simulink library "SUB_ECU_L4_MABX_HW_Interface"  (R2018a)
settings: Solver=VariableStepAuto  StartTime=0.0  StopTime=10.0  RelTol=1e-3
PostLoadFcn:
  | , if any(exist('dsrtsu_mdlpostloadfcn', 'file') == [2, 3, 6]), try dsrtsu_mdlpostloadfcn('Execute', bdroot); catch fprintf('Error in PostLoadFcn (dsrtsu_mdlpostloadfcn) for model "%s":\n %s\n', bdroot, lasterr); end, end,
undefined symbols (not defined in the file or in its folder): CANR_PROPB_REAX_3_13_CHANNEL_APV, CANR_PROPB_REAX_4_13_CHANNEL_APV, CANR_PROPB_XPR_1_50_CHANNEL_APV, ENUM_CAN_RX_T, ENUM_CAN_TX_T, ENUM_REAX_OPERATION_MODE_T, ENUM_SIGNAL_HEALTH_T, ENUM_XBR_CONTROL_MODE_T, ENUM_XBR_EBI_MODE_T, ENUM_XBR_PASS_THROUGH_ACTIVE_T, ENUM_XBR_PRIORITY_T, ENUM_XPR_INHIBIT_PARK_MANUAL_T, ENUM_XPR_INHIBIT_UNPARK_MANUAL_T, ENUM_XPR_PARK_MANUAL_T, ENUM_XPR_UNPARK_MANUAL_T, PROPB_REAX_1_E4_DES_POS_SIG_SRC_APV, PROPB_REAX_1_E4_DESIRED_OPMODE_APV, PROPB_REAX_1_E4_DESIRED_POSITION_APV, ptc_matlab_lib
libraries: PTC_MBDS_LIB x264, rtican x172, EmE_MBD_Blockset x39, simulink x34, $bdroot x16, rti1401lib_dio_type4 x8, simulink_need_slupdate x7, dsa_tcpip_lib x4, rti1401lib_adc_type4 x3, rtmapslib x3, rtitasklib x3
(part 51 of 51)

== system SUB_ECU_L4_MABX_HW_Interface/DIGITAL/PWM pedal input management/Diagnose pedal input signals/Leaky_bucket1 ==
  Signal_valid_range_max : Inport
  Signal_valid_range_min : Inport  Port=2
  Count_Max : Inport  Port=3
  Count_Min : Inport  Port=4
  Input_signal : Inport  Port=5
  Check Dynamic Range1 : simulink/Model Verification/Check  Dynamic Range  Description=min < u < max  enabled=on  stopWhenAssertionFail=off  export=on  icon=graphic
      settings: SourceProductName=Simulink  SourceProductBaseCode=SL
  Decrement Real World3 : simulink/Additional Math & Discrete/Additional Math: Increment - Decrement/Decrement Real World
      settings: SourceProductName=Simulink  SourceProductBaseCode=SL
  Dynamic_saturation3 : EmE_MBD_Blockset/Discontinuities/Dynamic_saturation
      settings: SourceProductName=PACCAR EmE MBD Blockset
  If_Then_Else3 : EmE_MBD_Blockset/Signal Routing/If_Then_Else
      settings: SourceProductName=PACCAR EmE MBD Blockset
  Increment Real World3 : simulink/Additional Math & Discrete/Additional Math: Increment - Decrement/Increment Real World
      settings: SourceProductName=Simulink  SourceProductBaseCode=SL
  Relational Operator8 : RelationalOperator  Operator=<=  OutDataTypeStr=boolean  RndMeth=Nearest
  Relational Operator9 : RelationalOperator  Operator=~=  OutDataTypeStr=boolean  RndMeth=Nearest
  Unit Delay External IC3 : simulink_need_slupdate/Unit Delay External IC  tsamp=-1
      settings: SourceProductName=Simulink  SourceProductBaseCode=SL
  Fault_Count : Outport
  F_Fault_Soft : Outport  Port=2
  F_Fault_Hard : Outport  Port=3
  wires:
  Count_Min/1 -> Unit Delay External IC3/2, Relational Operator9/2, Dynamic_saturation3/3
  Dynamic_saturation3/1 -> Relational Operator9/1, Unit Delay External IC3/1, Fault_Count/1, Relational Operator8/2  "Fault_Count"
  Decrement Real World3/1 -> If_Then_Else3/2
  Increment Real World3/1 -> If_Then_Else3/3
  Relational Operator9/1 -> F_Fault_Soft/1  "F_Fault_Soft"
  Input_signal/1 -> Check Dynamic Range1/3
  Unit Delay External IC3/1 -> Increment Real World3/1, Decrement Real World3/1
  Count_Max/1 -> Relational Operator8/1, Dynamic_saturation3/1
  Relational Operator8/1 -> F_Fault_Hard/1  "F_Fault_Hard"
  Signal_valid_range_max/1 -> Check Dynamic Range1/1
  Check Dynamic Range1/1 -> If_Then_Else3/1  "f_signal_valid"
  Signal_valid_range_min/1 -> Check Dynamic Range1/2
  If_Then_Else3/1 -> Dynamic_saturation3/2

== system SUB_ECU_L4_MABX_HW_Interface/DIGITAL/PWM pedal input management/Diagnose pedal input signals/Leaky_bucket2 ==
  Signal_valid_range_max : Inport
  Signal_valid_range_min : Inport  Port=2
  Count_Max : Inport  Port=3
  Count_Min : Inport  Port=4
  Input_signal : Inport  Port=5
  Check Dynamic Range1 : simulink/Model Verification/Check  Dynamic Range  Description=min < u < max  enabled=on  stopWhenAssertionFail=off  export=on  icon=graphic
      settings: SourceProductName=Simulink  SourceProductBaseCode=SL
  Decrement Real World3 : simulink/Additional Math & Discrete/Additional Math: Increment - Decrement/Decrement Real World
      settings: SourceProductName=Simulink  SourceProductBaseCode=SL
  Dynamic_saturation3 : EmE_MBD_Blockset/Discontinuities/Dynamic_saturation
      settings: SourceProductName=PACCAR EmE MBD Blockset
  If_Then_Else3 : EmE_MBD_Blockset/Signal Routing/If_Then_Else
      settings: SourceProductName=PACCAR EmE MBD Blockset
  Increment Real World3 : simulink/Additional Math & Discrete/Additional Math: Increment - Decrement/Increment Real World
      settings: SourceProductName=Simulink  SourceProductBaseCode=SL
  Relational Operator8 : RelationalOperator  Operator=<=  OutDataTypeStr=boolean  RndMeth=Nearest
  Relational Operator9 : RelationalOperator  Operator=~=  OutDataTypeStr=boolean  RndMeth=Nearest
  Unit Delay External IC3 : simulink_need_slupdate/Unit Delay External IC  tsamp=-1
      settings: SourceProductName=Simulink  SourceProductBaseCode=SL
  Fault_Count : Outport
  F_Fault_Soft : Outport  Port=2
  F_Fault_Hard : Outport  Port=3
  wires:
  Count_Min/1 -> Unit Delay External IC3/2, Relational Operator9/2, Dynamic_saturation3/3
  Dynamic_saturation3/1 -> Relational Operator9/1, Unit Delay External IC3/1, Fault_Count/1, Relational Operator8/2  "Fault_Count"
  Decrement Real World3/1 -> If_Then_Else3/2
  Increment Real World3/1 -> If_Then_Else3/3
  Relational Operator9/1 -> F_Fault_Soft/1  "F_Fault_Soft"
  Input_signal/1 -> Check Dynamic Range1/3
  Unit Delay External IC3/1 -> Increment Real World3/1, Decrement Real World3/1
  Count_Max/1 -> Relational Operator8/1, Dynamic_saturation3/1
  Relational Operator8/1 -> F_Fault_Hard/1  "F_Fault_Hard"
  Signal_valid_range_max/1 -> Check Dynamic Range1/1
  Check Dynamic Range1/1 -> If_Then_Else3/1  "f_signal_valid"
  Signal_valid_range_min/1 -> Check Dynamic Range1/2
  If_Then_Else3/1 -> Dynamic_saturation3/2

== system SUB_ECU_L4_MABX_HW_Interface/DIGITAL/PWM pedal input management/Diagnose pedal input signals/Leaky_bucket3 ==
  Signal_valid_range_max : Inport
  Signal_valid_range_min : Inport  Port=2
  Count_Max : Inport  Port=3
  Count_Min : Inport  Port=4
  Input_signal : Inport  Port=5
  Check Dynamic Range1 : simulink/Model Verification/Check  Dynamic Range  Description=min < u < max  enabled=on  stopWhenAssertionFail=off  export=on  icon=graphic
      settings: SourceProductName=Simulink  SourceProductBaseCode=SL
  Decrement Real World3 : simulink/Additional Math & Discrete/Additional Math: Increment - Decrement/Decrement Real World
      settings: SourceProductName=Simulink  SourceProductBaseCode=SL
  Dynamic_saturation3 : EmE_MBD_Blockset/Discontinuities/Dynamic_saturation
      settings: SourceProductName=PACCAR EmE MBD Blockset
  If_Then_Else3 : EmE_MBD_Blockset/Signal Routing/If_Then_Else
      settings: SourceProductName=PACCAR EmE MBD Blockset
  Increment Real World3 : simulink/Additional Math & Discrete/Additional Math: Increment - Decrement/Increment Real World
      settings: SourceProductName=Simulink  SourceProductBaseCode=SL
  Relational Operator8 : RelationalOperator  Operator=<=  OutDataTypeStr=boolean  RndMeth=Nearest
  Relational Operator9 : RelationalOperator  Operator=~=  OutDataTypeStr=boolean  RndMeth=Nearest
  Unit Delay External IC3 : simulink_need_slupdate/Unit Delay External IC  tsamp=-1
      settings: SourceProductName=Simulink  SourceProductBaseCode=SL
  Fault_Count : Outport
  F_Fault_Soft : Outport  Port=2
  F_Fault_Hard : Outport  Port=3
  wires:
  If_Then_Else3/1 -> Dynamic_saturation3/2
  Signal_valid_range_min/1 -> Check Dynamic Range1/2
  Check Dynamic Range1/1 -> If_Then_Else3/1  "f_signal_valid"
  Signal_valid_range_max/1 -> Check Dynamic Range1/1
  Relational Operator8/1 -> F_Fault_Hard/1  "F_Fault_Hard"
  Count_Max/1 -> Dynamic_saturation3/1, Relational Operator8/1
  Unit Delay External IC3/1 -> Decrement Real World3/1, Increment Real World3/1
  Input_signal/1 -> Check Dynamic Range1/3
  Relational Operator9/1 -> F_Fault_Soft/1  "F_Fault_Soft"
  Increment Real World3/1 -> If_Then_Else3/3
  Decrement Real World3/1 -> If_Then_Else3/2
  Dynamic_saturation3/1 -> Relational Operator8/2, Fault_Count/1, Unit Delay External IC3/1, Relational Operator9/1  "Fault_Count"
  Count_Min/1 -> Dynamic_saturation3/3, Relational Operator9/2, Unit Delay External IC3/2

== system SUB_ECU_L4_MABX_HW_Interface/DIGITAL/PWM pedal input management/Diagnose pedal input signals/Leaky_bucket4 ==
  Signal_valid_range_max : Inport
  Signal_valid_range_min : Inport  Port=2
  Count_Max : Inport  Port=3
  Count_Min : Inport  Port=4
  Input_signal : Inport  Port=5
  Check Dynamic Range1 : simulink/Model Verification/Check  Dynamic Range  Description=min < u < max  enabled=on  stopWhenAssertionFail=off  export=on  icon=graphic
      settings: SourceProductName=Simulink  SourceProductBaseCode=SL
  Decrement Real World3 : simulink/Additional Math & Discrete/Additional Math: Increment - Decrement/Decrement Real World
      settings: SourceProductName=Simulink  SourceProductBaseCode=SL
  Dynamic_saturation3 : EmE_MBD_Blockset/Discontinuities/Dynamic_saturation
      settings: SourceProductName=PACCAR EmE MBD Blockset
  If_Then_Else3 : EmE_MBD_Blockset/Signal Routing/If_Then_Else
      settings: SourceProductName=PACCAR EmE MBD Blockset
  Increment Real World3 : simulink/Additional Math & Discrete/Additional Math: Increment - Decrement/Increment Real World
      settings: SourceProductName=Simulink  SourceProductBaseCode=SL
  Relational Operator8 : RelationalOperator  Operator=<=  OutDataTypeStr=boolean  RndMeth=Nearest
  Relational Operator9 : RelationalOperator  Operator=~=  OutDataTypeStr=boolean  RndMeth=Nearest
  Unit Delay External IC3 : simulink_need_slupdate/Unit Delay External IC  tsamp=-1
      settings: SourceProductName=Simulink  SourceProductBaseCode=SL
  Fault_Count : Outport
  F_Fault_Soft : Outport  Port=2
  F_Fault_Hard : Outport  Port=3
  wires:
  If_Then_Else3/1 -> Dynamic_saturation3/2
  Signal_valid_range_min/1 -> Check Dynamic Range1/2
  Check Dynamic Range1/1 -> If_Then_Else3/1  "f_signal_valid"
  Signal_valid_range_max/1 -> Check Dynamic Range1/1
  Relational Operator8/1 -> F_Fault_Hard/1  "F_Fault_Hard"
  Count_Max/1 -> Dynamic_saturation3/1, Relational Operator8/1
  Unit Delay External IC3/1 -> Decrement Real World3/1, Increment Real World3/1
  Input_signal/1 -> Check Dynamic Range1/3
  Relational Operator9/1 -> F_Fault_Soft/1  "F_Fault_Soft"
  Increment Real World3/1 -> If_Then_Else3/3
  Decrement Real World3/1 -> If_Then_Else3/2
  Dynamic_saturation3/1 -> Relational Operator8/2, Fault_Count/1, Unit Delay External IC3/1, Relational Operator9/1  "Fault_Count"
  Count_Min/1 -> Dynamic_saturation3/3, Relational Operator9/2, Unit Delay External IC3/2

== system SUB_ECU_L4_MABX_HW_Interface/CAN_Out_PTC_1571/CAN_TX_10ms/Encode_PROPB_REAX_1/PropB_REAX_1_E4_CommandFromExternalController/ALL_CTRL_DISABLED ==
  Enable : EnablePort
      settings: AttributesFormatString=States when enabling: %<StatesWhenEnabling>
  Constant : Constant  Value=typecast(uint32(hex2dec('FFFFFFFF')), 'int32')
  Out1 : Outport  InitialOutput=0
      settings: AttributesFormatString=Output when disabled: %<OutputWhenDisabled>
  wires:
  Constant/1 -> Out1/1

== system SUB_ECU_L4_MABX_HW_Interface/CAN_Out_PTC_1571/CAN_TX_10ms/Encode_PROPB_REAX_1/PropB_REAX_1_E4_CommandFromExternalController/DEFAULT_TRQ_CTRL_MODE ==
  Enable : EnablePort
      settings: AttributesFormatString=States when enabling: %<StatesWhenEnabling>
  Constant : Constant  Value=typecast(uint32(hex2dec('FFFFFFFF')), 'int32')
  Out1 : Outport  InitialOutput=0
      settings: AttributesFormatString=Output when disabled: %<OutputWhenDisabled>
  wires:
  Constant/1 -> Out1/1

== system SUB_ECU_L4_MABX_HW_Interface/CAN_Out_PTC_1571/CAN_TX_10ms/Encode_PROPB_REAX_1/PropB_REAX_1_E4_CommandFromExternalController/Desired_Steering_Angle ==
  DesiredSteeringAngle : Inport
  OperatorEnable : Inport  Port=2
  Constant1 : Constant  Value=PROPB_REAX_1_E4_DES_POS_SIG_SRC_APV
  Constant7 : Constant  Value=PROPB_REAX_1_E4_DESIRED_POSITION_APV
  Multiport_Switch : MultiPortSwitch  DataPortOrder=Specify indices  DataPortIndices={ENUM_STEERING_POS_SIGNAL_SOURCE_T.SW_EMULATION, ENUM_STEERING_POS_SIGNAL_SOURCE_T.ESTIMATION}  DataPortForDefault=Additional data port  SaturateOnIntegerOverflow=on  InputSameDT=on
      settings: AttributesFormatString=Zero-based indexing: %<zeroidx>
  Switch : Switch  Criteria=u2 ~= 0
  zero : Constant  Value=0
  Out1 : Outport
  wires:
  zero/1 -> Switch/3
  Switch/1 -> Out1/1
  OperatorEnable/1 -> Switch/2
  Multiport_Switch/1 -> Switch/1
  DesiredSteeringAngle/1 -> Multiport_Switch/3
  Constant7/1 -> Multiport_Switch/2, Multiport_Switch/4
  Constant1/1 -> Multiport_Switch/1

== system SUB_ECU_L4_MABX_HW_Interface/CAN_Out_PTC_1571/CAN_TX_10ms/Encode_PROPB_REAX_1/PropB_REAX_1_E4_CommandFromExternalController/EXT_TRQ_CTRL_MODE_A ==
  Enable : EnablePort
      settings: AttributesFormatString=States when enabling: %<StatesWhenEnabling>
  Constant : Constant  Value=typecast(uint32(hex2dec('FFFFFFFF')), 'int32')
  Out1 : Outport  InitialOutput=0
      settings: AttributesFormatString=Output when disabled: %<OutputWhenDisabled>
  wires:
  Constant/1 -> Out1/1

== system SUB_ECU_L4_MABX_HW_Interface/CAN_Out_PTC_1571/CAN_TX_10ms/Encode_PROPB_REAX_1/PropB_REAX_1_E4_CommandFromExternalController/EXT_TRQ_CTRL_MODE_B ==
  Enable : EnablePort
      settings: AttributesFormatString=States when enabling: %<StatesWhenEnabling>
  Constant : Constant  Value=typecast(uint32(hex2dec('FFFFFFFF')), 'int32')
  Out1 : Outport  InitialOutput=0
      settings: AttributesFormatString=Output when disabled: %<OutputWhenDisabled>
  wires:
  Constant/1 -> Out1/1

== system SUB_ECU_L4_MABX_HW_Interface/CAN_Out_PTC_1571/CAN_TX_10ms/Encode_PROPB_REAX_1/PropB_REAX_1_E4_CommandFromExternalController/EXT_TRQ_CTRL_MODE_C ==
  Enable : EnablePort
      settings: AttributesFormatString=States when enabling: %<StatesWhenEnabling>
  Constant : Constant  Value=typecast(uint32(hex2dec('FFFFFFFF')), 'int32')
  Out1 : Outport  InitialOutput=0
      settings: AttributesFormatString=Output when disabled: %<OutputWhenDisabled>
  wires:
  Constant/1 -> Out1/1

== system SUB_ECU_L4_MABX_HW_Interface/CAN_Out_PTC_1571/CAN_TX_10ms/Encode_PROPB_REAX_1/PropB_REAX_1_E4_CommandFromExternalController/POSITION_CONTROL_MODE ==
  In1 : Inport
  Enable : EnablePort
      settings: AttributesFormatString=States when enabling: %<StatesWhenEnabling>
  Constant : Constant  Value=8192/360
  Data Type Conversion : DataTypeConversion  OutDataTypeStr=int32  SaturateOnIntegerOverflow=on
  Product : Product  Inputs=**  OutDataTypeStr=Inherit: Inherit via back propagation  SaturateOnIntegerOverflow=on  InputSameDT=on
      settings: AttributesFormatString=Saturate: %<SaturateOnIntegerOverflow>
  Out1 : Outport  InitialOutput=0
      settings: AttributesFormatString=Output when disabled: %<OutputWhenDisabled>
  wires:
  Data Type Conversion/1 -> Out1/1
  Product/1 -> Data Type Conversion/1
  Constant/1 -> Product/2
  In1/1 -> Product/1

== matlab function SUB_ECU_L4_MABX_HW_Interface/CAN_Truck166/CAN_RX_EC1_00/CAN_RX_EC1_00/serialize_tpdt ==
  data: RX_status output boolean; data_packet_previous input uint8; Data output uint8; TotalNumberOfPackets input uint8; SequenceNumber input uint8; byte1 input uint8; byte2 input uint8; byte3 input uint8; byte4 input uint8; byte5 input uint8; byte6 input uint8; byte7 input uint8
function [RX_status, Data] = serialize_tpdt(data_packet_previous, ...
    TotalNumberOfPackets, ...
    SequenceNumber, byte1, byte2, byte3, byte4, byte5, byte6, byte7)
%#codegen

if SequenceNumber > 1
    Data = data_packet_previous;
else
    Data = uint8(255) * ones(39, 1, 'uint8');
end
starting_index = 7*SequenceNumber - 6;
Data(starting_index : starting_index + 6) = [byte1; byte2; byte3; byte4; byte5; byte6; byte7];
RX_status = (SequenceNumber == TotalNumberOfPackets);

end

== matlab function SUB_ECU_L4_MABX_HW_Interface/CAN_Truck1571/CAN_RX_EC1_00/CAN_RX_EC1_00/serialize_tpdt ==
  data: RX_status output boolean; data_packet_previous input uint8; Data output uint8; TotalNumberOfPackets input uint8; SequenceNumber input uint8; byte1 input uint8; byte2 input uint8; byte3 input uint8; byte4 input uint8; byte5 input uint8; byte6 input uint8; byte7 input uint8
function [RX_status, Data] = serialize_tpdt(data_packet_previous, ...
    TotalNumberOfPackets, ...
    SequenceNumber, byte1, byte2, byte3, byte4, byte5, byte6, byte7)
%#codegen

if SequenceNumber > 1
    Data = data_packet_previous;
else
    Data = uint8(255) * ones(39, 1, 'uint8');
end
starting_index = 7*SequenceNumber - 6;
Data(starting_index : starting_index + 6) = [byte1; byte2; byte3; byte4; byte5; byte6; byte7];
RX_status = (SequenceNumber == TotalNumberOfPackets);

end

== matlab function SUB_ECU_L4_MABX_HW_Interface/CAN_Truck1571/CAN_RX_VI_00/CAN_RX_VI_00/serialize_tpdt ==
  data: RX_status output boolean; data_packet_previous input uint8; Data output uint8; TotalNumberOfPackets input uint8; SequenceNumber input uint8; byte1 input uint8; byte2 input uint8; byte3 input uint8; byte4 input uint8; byte5 input uint8; byte6 input uint8; byte7 input uint8
function [RX_status, Data] = serialize_tpdt(data_packet_previous, ...
    TotalNumberOfPackets, ...
    SequenceNumber, byte1, byte2, byte3, byte4, byte5, byte6, byte7)
%#codegen

if SequenceNumber > 1
    Data = data_packet_previous;
else
    Data = uint8(255) * ones(17, 1, 'uint8');
end
starting_index = 7*SequenceNumber - 6;
Data(starting_index : starting_index + 6) = [byte1; byte2; byte3; byte4; byte5; byte6; byte7];
RX_status = (SequenceNumber == TotalNumberOfPackets);

end

== stateflow chart SUB_ECU_L4_MABX_HW_Interface/CAN_Out_PTC_1571/CAN_TX_BAM/Chart ==
  state Init
    en:State= uint8(0);
    en:enTPCM=logical(0);
    en:enTPDT=logical(0);
    en:TPCM_ts_Prev=TPCM_ts;
    en:TPDT_ts_Prev=TPDT_ts;
    en:TPDT_count=uint8(0);
  state StartMsg
    en:State= uint8(1);
    en:TPDT_count=uint8(1);
  state SendTPCM
    en:State=uint8(2);
    en:enTPCM=logical(1);
  state InterframeDelay
    en:State=uint8(3);
    en:enTPCM=logical(0);
    en:TPCM_ts_Prev=TPCM_ts;
  state SendTPDT
    en:State=uint8(4);
    en:enTPDT=logical(1);
  state InterframeDelay1
    en:State= uint8(5);
    en:enTPDT=logical(0);
    en:TPDT_ts_Prev=TPDT_ts;
  state CheckPacketCount
    en:State=uint8(6);
    en:TPDT_count=TPDT_count+uint8(1);
  state WaitForNextPeriod
    en:State=uint8(7);
  (default) -> Init
  Init -> StartMsg
  WaitForNextPeriod -> StartMsg : after(1.85,sec)
  StartMsg -> SendTPCM
  SendTPCM -> InterframeDelay : after(.010,sec)
  InterframeDelay -> SendTPDT : after(0.05, sec)
  CheckPacketCount -> SendTPDT [order 1] : [TPDT_count<=TPDT_total]
  SendTPDT -> InterframeDelay1 : after(0.01,sec)
  InterframeDelay1 -> CheckPacketCount : after(0.05,sec)
  CheckPacketCount -> WaitForNextPeriod [order 2]
  data: State output uint8; enTPDT output boolean; enTPCM output boolean; TPCM_ts input; TPDT_ts input; TPCM_ts_Prev output; TPDT_ts_Prev output; TPDT_count output uint8; TPDT_total input uint8

== stateflow chart SUB_ECU_L4_MABX_HW_Interface/DIGITAL/RationalityCheck/Chart ==
  state init
    en:DiagPassed=logical(0);
  state SwitchOff
  state SwitchOn
  state DiagPassed
    en:DiagPassed=logical(1);
  (default) -> init
  init -> SwitchOn [order 2] : [Input==1]
  init -> SwitchOff [order 1] : [Input==0]
  SwitchOff -> DiagPassed : [Input==1]
  SwitchOn -> SwitchOff : [Input==0]
  data: Input input boolean; DiagPassed output boolean

== stateflow chart SUB_ECU_L4_MABX_HW_Interface/DIGITAL/PWM pedal input management/Diagnose pedal input signals/Health State Machine PWM Sensor 1 ==
  state NO_FAILURE
    en: Pedal_1_pwm_health_state = ENUM_SIGNAL_HEALTH_T.FAULT_INACTIVE;
  state FAILURE_DETECTED
    state PENDING
      en: Pedal_1_pwm_health_state = ENUM_SIGNAL_HEALTH_T.FAULT_PENDING;
    state ERROR
      en: Pedal_1_pwm_health_state = ENUM_SIGNAL_HEALTH_T.FAULT_ACTIVE;
    (default) -> PENDING
    PENDING -> ERROR [order 2] : [F_Pedal_1_pwm_fault_active]
    ERROR -> PENDING : [~F_Pedal_1_pwm_fault_active]
  (default) -> NO_FAILURE
  NO_FAILURE -> FAILURE_DETECTED : [F_Pedal_1_pwm_fault_pending || ...
      | F_Pedal_1_pwm_fault_active]
  PENDING -> NO_FAILURE [order 1] : [~F_Pedal_1_pwm_fault_pending && ...
      | ~F_Pedal_1_pwm_fault_active]
  data: F_Pedal_1_pwm_fault_pending input; F_Pedal_1_pwm_fault_active input; Pedal_1_pwm_health_state output Enum: ENUM_SIGNAL_HEALTH_T

== stateflow chart SUB_ECU_L4_MABX_HW_Interface/DIGITAL/PWM pedal input management/Diagnose pedal input signals/Health State Machine PWM Sensor 2 ==
  state NO_FAILURE
    en: Pedal_2_pwm_health_state = ENUM_SIGNAL_HEALTH_T.FAULT_INACTIVE;
  state FAILURE_DETECTED
    state PENDING
      en: Pedal_2_pwm_health_state = ENUM_SIGNAL_HEALTH_T.FAULT_PENDING;
    state ERROR
      en: Pedal_2_pwm_health_state = ENUM_SIGNAL_HEALTH_T.FAULT_ACTIVE;
    (default) -> PENDING
    PENDING -> ERROR [order 2] : [F_Pedal_2_pwm_fault_active]
    ERROR -> PENDING : [~F_Pedal_2_pwm_fault_active]
  (default) -> NO_FAILURE
  NO_FAILURE -> FAILURE_DETECTED : [F_Pedal_2_pwm_fault_pending || ...
      | F_Pedal_2_pwm_fault_active]
  PENDING -> NO_FAILURE [order 1] : [~F_Pedal_2_pwm_fault_pending && ...
      | ~F_Pedal_2_pwm_fault_active]
  data: F_Pedal_2_pwm_fault_pending input; F_Pedal_2_pwm_fault_active input; Pedal_2_pwm_health_state output

== matlab function SUB_ECU_L4_MABX_HW_Interface/CAN_Truck166/CAN_RX_VI_00/CAN_RX_VI_00/serialize_tpdt ==
  data: RX_status output boolean; data_packet_previous input uint8; Data output uint8; TotalNumberOfPackets input uint8; SequenceNumber input uint8; byte1 input uint8; byte2 input uint8; byte3 input uint8; byte4 input uint8; byte5 input uint8; byte6 input uint8; byte7 input uint8
function [RX_status, Data] = serialize_tpdt(data_packet_previous, ...
    TotalNumberOfPackets, ...
    SequenceNumber, byte1, byte2, byte3, byte4, byte5, byte6, byte7)
%#codegen

if SequenceNumber > 1
    Data = data_packet_previous;
else
    Data = uint8(255) * ones(17, 1, 'uint8');
end
starting_index = 7*SequenceNumber - 6;
Data(starting_index : starting_index + 6) = [byte1; byte2; byte3; byte4; byte5; byte6; byte7];
RX_status = (SequenceNumber == TotalNumberOfPackets);

end

== matlab function SUB_ECU_L4_MABX_HW_Interface/CAN_PIC_KW/CAN_RX_EC1_00/CAN_RX_EC1_00/serialize_tpdt ==
  data: RX_status output boolean; data_packet_previous input uint8; Data output uint8; TotalNumberOfPackets input uint8; SequenceNumber input uint8; byte1 input uint8; byte2 input uint8; byte3 input uint8; byte4 input uint8; byte5 input uint8; byte6 input uint8; byte7 input uint8
function [RX_status, Data] = serialize_tpdt(data_packet_previous, ...
    TotalNumberOfPackets, ...
    SequenceNumber, byte1, byte2, byte3, byte4, byte5, byte6, byte7)
%#codegen

if SequenceNumber > 1
    Data = data_packet_previous;
else
    Data = uint8(255) * ones(39, 1, 'uint8');
end
starting_index = 7*SequenceNumber - 6;
Data(starting_index : starting_index + 6) = [byte1; byte2; byte3; byte4; byte5; byte6; byte7];
RX_status = (SequenceNumber == TotalNumberOfPackets);

end

== matlab function SUB_ECU_L4_MABX_HW_Interface/CAN_PIC_KW/CAN_RX_VI_00/CAN_RX_VI_00/serialize_tpdt ==
  data: RX_status output boolean; data_packet_previous input uint8; Data output uint8; TotalNumberOfPackets input uint8; SequenceNumber input uint8; byte1 input uint8; byte2 input uint8; byte3 input uint8; byte4 input uint8; byte5 input uint8; byte6 input uint8; byte7 input uint8
function [RX_status, Data] = serialize_tpdt(data_packet_previous, ...
    TotalNumberOfPackets, ...
    SequenceNumber, byte1, byte2, byte3, byte4, byte5, byte6, byte7)
%#codegen

if SequenceNumber > 1
    Data = data_packet_previous;
else
    Data = uint8(255) * ones(17, 1, 'uint8');
end
starting_index = 7*SequenceNumber - 6;
Data(starting_index : starting_index + 6) = [byte1; byte2; byte3; byte4; byte5; byte6; byte7];
RX_status = (SequenceNumber == TotalNumberOfPackets);

end
